simulink library "lib_serial"  (R2022b)
settings: Solver=VariableStepAuto  StartTime=0.0  StopTime=10.0  RelTol=1e-3
settings Model: Creator=F64236C  LastModifiedBy=F64236C

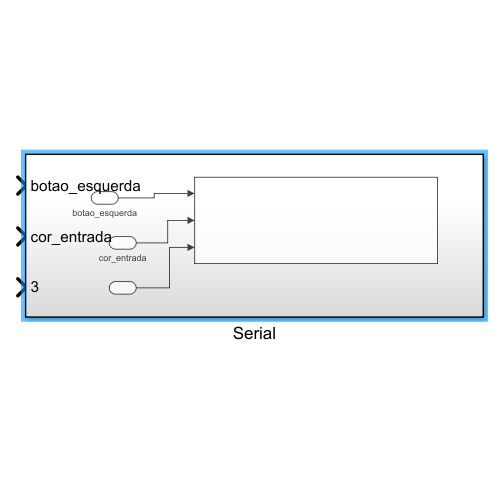
[thumbnail: Simulink's stored preview of the top-level diagram]
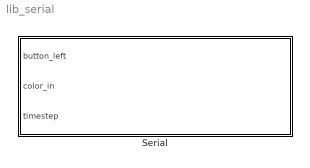
== system lib_serial ==
  Serial : Subsystem

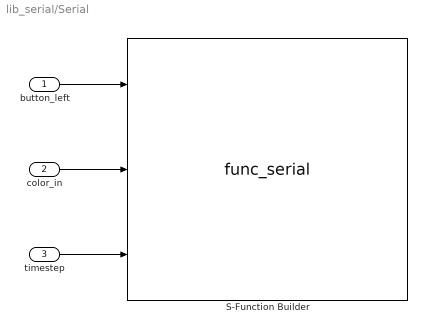
== system lib_serial/Serial ==
  button_left : Inport
  color_in : Inport  Port=2
  timestep : Inport  Port=3
  S-Function Builder : S-Function  FunctionName=func_serial  SFunctionModules=func_serial_wrapper.cpp  SFunctionDeploymentMode=off  EnableBusSupport=off  mask(S-Function Builder){}
      mask help: Simulink:masks:SFunctionBuilder_MD
      mask init:
      | val = [[.9  0.75 0.75 1 1 .9 .9 1]',[1 1 0.75 0.75 .9 .9 1 .9]'];try , sys = get_param(gcb,'SfunBuilderFcnName');if isempty(sys), sys = get_param(gcb,'FunctionName'); end,catch, sys = get_param(gcb,'FunctionName'); end
      settings: CopyFcn=set_param(gcbh,'LinkStatus','none')  OpenFcn=sfunctionwizard(gcbh)
      mask Display:
      | plot(val(:,1),val(:,2))
      | disp(sys)
      | port_label('input',1,'button_left')
      | port_label('input',2,'color_in')
      | port_label('input',3,'timestep')
  wires:
  color_in/1 -> S-Function Builder/2
  button_left/1 -> S-Function Builder/1
  timestep/1 -> S-Function Builder/3
